simulink subsystem "station2a"  (R2024b)
settings: Solver=VariableStepAuto  StartTime=0.0  StopTime=10.0  RelTol=1e-3
undefined symbols (not defined in the file): DiscIntNeverNeededParam, h, R3, ResistanceM, Rt4, Ts, Zm
libraries: ee_lib x105, nesl_utility x83, fl_lib x73, simulink x6, simetran x1, powerlib_extras x1
(part 2 of 4)

== system station2a/Filters 60Hz4 ==
  s : Inport
  Circuit Breaker (Three-Phase) : ee_lib/Switches & Breakers/Circuit Breaker (Three-Phase)  R_closed=0.001 Ohm  G_open=1e-6 1/Ohm  threshold=0.5 V  breaker_behavior=ee.enum.switches.breakerBehavior.zeroCrossingEnable
      settings: InternalSimscapePortConfiguration="{\"Bottom\":[],\"Left\":[{\"id\":\"vT\",\"label\":\"vT\",\"type\":\"input\"},{\"id\":\"N1\",\"label\":\"~1\",\"type\":\"foundation.electrical.three_phase\"}],\"Right\":[{\"id\":\"N2\",\"label\":\"~2\",\"type\":\"foundation.electrical.three_phase\"}],\"Top\":[]}"
  Constant : Constant
  Electrical Reference : fl_lib/Electrical/Electrical Elements/Electrical Reference
  Simulink-PS Converter : nesl_utility/Simulink-PS Converter  PhysicalDomain=network_engine_domain  SubClassName=ps_input  LeftPortType=input  RightPortType=output  PseudoPeriodic=off  Frequencies=[]  NoiseDistribution=none  NoiseParameters=[]  Unit=1  AffineConversion=off  FilteringAndDerivatives=provide  SimscapeFilterOrder=1  InputFilterTimeConstant=0.001  UdotUserProvided=0
  Sum : Sum  Inputs=|-+
  Wye-Connected Load : ee_lib/Passive/RLC Assemblies/Wye-Connected Load  port_option=ee.enum.threePhasePort.composite  parameterization=ee.enum.rlc.parameterization.ratedpower  component_structure=ee.enum.rlc.structure.R  component_structure_PQ=ee.enum.rlc.structure.C  R=1 Ohm  L=1e-3 H  C=1e-6 F  VRated=345e3 V  FRated=50 Hz  P=1e3 W  Qpos=1e2 A*V  Qneg=-150e6/4 A*V  R_parasitic=1e-6 Ohm  G_parasitic=1e-6 1/Ohm  R_parasitic_PQ=0 Ohm  G_parasitic_PQ=1e-6 1/Ohm  Vmag0=500e3 V  Vang0=0 deg  Freq0=60 Hz  IL_specify=off  IL_priority=High  IL=[0, 0, 0] A  IL_nominal_specify=off  IL_nominal_value=1  IL_nominal_unit=A  VC_specify=off  VC_priority=High  VC=[0, 0, 0] V  VC_nominal_specify=off  VC_nominal_value=1  VC_nominal_unit=V
  high-pass filter : ee_lib/Passive/Passive Harmonic Filter (Three-Phase)  QRated=150e6/4 A*V  VRated=345e3 V  FRated=50 Hz  qfactor=3  type_option=ee.enum.filtertype.HPsecondorder  connection_option=ee.enum.filterconnection.Yg  ftuned=24 * 24 Hz  ftuned1=7 * 60 Hz  ftuned2=11 * 60 Hz  I_specify=off  I_priority=None  I=[0, 0, 0] A  I_nominal_specify=off  I_nominal_value=1  I_nominal_unit=A  V_specify=off  V_priority=None  V=[0, 0, 0] V  V_nominal_specify=off  V_nominal_value=1  V_nominal_unit=V
      settings: InternalSimscapePortConfiguration="{\"Bottom\":[],\"Left\":[{\"id\":\"N\",\"label\":\"~\",\"type\":\"foundation.electrical.three_phase\"}],\"Right\":[],\"Top\":[]}"
  tuned flter 11th : ee_lib/Passive/Passive Harmonic Filter (Three-Phase)  QRated=150e6/4 A*V  VRated=345e3 V  FRated=50 Hz  qfactor=100  type_option=ee.enum.filtertype.BPsingle  connection_option=ee.enum.filterconnection.Yg  ftuned=11 * 50 Hz  ftuned1=7 * 60 Hz  ftuned2=11 * 60 Hz  I_specify=off  I_priority=None  I=[0, 0, 0] A  I_nominal_specify=off  I_nominal_value=1  I_nominal_unit=A  V_specify=off  V_priority=None  V=[0, 0, 0] V  V_nominal_specify=off  V_nominal_value=1  V_nominal_unit=V
      settings: InternalSimscapePortConfiguration="{\"Bottom\":[],\"Left\":[{\"id\":\"N\",\"label\":\"~\",\"type\":\"foundation.electrical.three_phase\"}],\"Right\":[],\"Top\":[]}"
  tuned flter 13th : ee_lib/Passive/Passive Harmonic Filter (Three-Phase)  QRated=150e6/4 A*V  VRated=345e3 V  FRated=50 Hz  qfactor=100  type_option=ee.enum.filtertype.BPsingle  connection_option=ee.enum.filterconnection.Yg  ftuned=13 * 50 Hz  ftuned1=7 * 60 Hz  ftuned2=11 * 60 Hz  I_specify=off  I_priority=None  I=[0, 0, 0] A  I_nominal_specify=off  I_nominal_value=1  I_nominal_unit=A  V_specify=off  V_priority=None  V=[0, 0, 0] V  V_nominal_specify=off  V_nominal_value=1  V_nominal_unit=V
      settings: InternalSimscapePortConfiguration="{\"Bottom\":[],\"Left\":[{\"id\":\"N\",\"label\":\"~\",\"type\":\"foundation.electrical.three_phase\"}],\"Right\":[],\"Top\":[]}"
  abc : PMIOPort  Side=Right
  wires:
  s/1 -> Sum/1
  Constant/1 -> Sum/2
  Sum/1 -> Simulink-PS Converter/1
  connections:
  Electrical Reference/LConn1 -- Wye-Connected Load/RConn1
  Wye-Connected Load/LConn1 -- high-pass filter/LConn1 -- tuned flter 13th/LConn1 -- Circuit Breaker (Three-Phase)/LConn2 -- tuned flter 11th/LConn1
  Circuit Breaker (Three-Phase)/RConn1 -- abc/RConn1
  Simulink-PS Converter/RConn1 -- Circuit Breaker (Three-Phase)/LConn1

== system station2a/Filters 60Hz5 ==
  s : Inport
  Circuit Breaker (Three-Phase) : ee_lib/Switches & Breakers/Circuit Breaker (Three-Phase)  R_closed=0.001 Ohm  G_open=1e-6 1/Ohm  threshold=0.5 V  breaker_behavior=ee.enum.switches.breakerBehavior.zeroCrossingEnable
      settings: InternalSimscapePortConfiguration="{\"Bottom\":[],\"Left\":[{\"id\":\"vT\",\"label\":\"vT\",\"type\":\"input\"},{\"id\":\"N1\",\"label\":\"~1\",\"type\":\"foundation.electrical.three_phase\"}],\"Right\":[{\"id\":\"N2\",\"label\":\"~2\",\"type\":\"foundation.electrical.three_phase\"}],\"Top\":[]}"
  Constant : Constant
  Electrical Reference : fl_lib/Electrical/Electrical Elements/Electrical Reference
  Simulink-PS Converter : nesl_utility/Simulink-PS Converter  PhysicalDomain=network_engine_domain  SubClassName=ps_input  LeftPortType=input  RightPortType=output  PseudoPeriodic=off  Frequencies=[]  NoiseDistribution=none  NoiseParameters=[]  Unit=1  AffineConversion=off  FilteringAndDerivatives=provide  SimscapeFilterOrder=1  InputFilterTimeConstant=0.001  UdotUserProvided=0
  Sum : Sum  Inputs=|-+
  Wye-Connected Load : ee_lib/Passive/RLC Assemblies/Wye-Connected Load  port_option=ee.enum.threePhasePort.composite  parameterization=ee.enum.rlc.parameterization.ratedpower  component_structure=ee.enum.rlc.structure.R  component_structure_PQ=ee.enum.rlc.structure.C  R=1 Ohm  L=1e-3 H  C=1e-6 F  VRated=345e3 V  FRated=50 Hz  P=1e3 W  Qpos=1e2 A*V  Qneg=-150e6/4 A*V  R_parasitic=1e-6 Ohm  G_parasitic=1e-6 1/Ohm  R_parasitic_PQ=0 Ohm  G_parasitic_PQ=1e-6 1/Ohm  Vmag0=500e3 V  Vang0=0 deg  Freq0=60 Hz  IL_specify=off  IL_priority=High  IL=[0, 0, 0] A  IL_nominal_specify=off  IL_nominal_value=1  IL_nominal_unit=A  VC_specify=off  VC_priority=High  VC=[0, 0, 0] V  VC_nominal_specify=off  VC_nominal_value=1  VC_nominal_unit=V
  high-pass filter : ee_lib/Passive/Passive Harmonic Filter (Three-Phase)  QRated=150e6/4 A*V  VRated=345e3 V  FRated=50 Hz  qfactor=3  type_option=ee.enum.filtertype.HPsecondorder  connection_option=ee.enum.filterconnection.Yg  ftuned=24 * 24 Hz  ftuned1=7 * 60 Hz  ftuned2=11 * 60 Hz  I_specify=off  I_priority=None  I=[0, 0, 0] A  I_nominal_specify=off  I_nominal_value=1  I_nominal_unit=A  V_specify=off  V_priority=None  V=[0, 0, 0] V  V_nominal_specify=off  V_nominal_value=1  V_nominal_unit=V
      settings: InternalSimscapePortConfiguration="{\"Bottom\":[],\"Left\":[{\"id\":\"N\",\"label\":\"~\",\"type\":\"foundation.electrical.three_phase\"}],\"Right\":[],\"Top\":[]}"
  tuned flter 11th : ee_lib/Passive/Passive Harmonic Filter (Three-Phase)  QRated=150e6/4 A*V  VRated=345e3 V  FRated=50 Hz  qfactor=100  type_option=ee.enum.filtertype.BPsingle  connection_option=ee.enum.filterconnection.Yg  ftuned=11 * 50 Hz  ftuned1=7 * 60 Hz  ftuned2=11 * 60 Hz  I_specify=off  I_priority=None  I=[0, 0, 0] A  I_nominal_specify=off  I_nominal_value=1  I_nominal_unit=A  V_specify=off  V_priority=None  V=[0, 0, 0] V  V_nominal_specify=off  V_nominal_value=1  V_nominal_unit=V
      settings: InternalSimscapePortConfiguration="{\"Bottom\":[],\"Left\":[{\"id\":\"N\",\"label\":\"~\",\"type\":\"foundation.electrical.three_phase\"}],\"Right\":[],\"Top\":[]}"
  tuned flter 13th : ee_lib/Passive/Passive Harmonic Filter (Three-Phase)  QRated=150e6/4 A*V  VRated=345e3 V  FRated=50 Hz  qfactor=100  type_option=ee.enum.filtertype.BPsingle  connection_option=ee.enum.filterconnection.Yg  ftuned=13 * 50 Hz  ftuned1=7 * 60 Hz  ftuned2=11 * 60 Hz  I_specify=off  I_priority=None  I=[0, 0, 0] A  I_nominal_specify=off  I_nominal_value=1  I_nominal_unit=A  V_specify=off  V_priority=None  V=[0, 0, 0] V  V_nominal_specify=off  V_nominal_value=1  V_nominal_unit=V
      settings: InternalSimscapePortConfiguration="{\"Bottom\":[],\"Left\":[{\"id\":\"N\",\"label\":\"~\",\"type\":\"foundation.electrical.three_phase\"}],\"Right\":[],\"Top\":[]}"
  abc : PMIOPort  Side=Right
  wires:
  Sum/1 -> Simulink-PS Converter/1
  Constant/1 -> Sum/2
  s/1 -> Sum/1
  connections:
  Simulink-PS Converter/RConn1 -- Circuit Breaker (Three-Phase)/LConn1
  Circuit Breaker (Three-Phase)/RConn1 -- abc/RConn1
  tuned flter 11th/LConn1 -- Circuit Breaker (Three-Phase)/LConn2 -- tuned flter 13th/LConn1 -- high-pass filter/LConn1 -- Wye-Connected Load/LConn1
  Electrical Reference/LConn1 -- Wye-Connected Load/RConn1

== system station2a/Filters 60Hz6 ==
  s : Inport
  Circuit Breaker (Three-Phase) : ee_lib/Switches & Breakers/Circuit Breaker (Three-Phase)  R_closed=0.001 Ohm  G_open=1e-6 1/Ohm  threshold=0.5 V  breaker_behavior=ee.enum.switches.breakerBehavior.zeroCrossingEnable
      settings: InternalSimscapePortConfiguration="{\"Bottom\":[],\"Left\":[{\"id\":\"vT\",\"label\":\"vT\",\"type\":\"input\"},{\"id\":\"N1\",\"label\":\"~1\",\"type\":\"foundation.electrical.three_phase\"}],\"Right\":[{\"id\":\"N2\",\"label\":\"~2\",\"type\":\"foundation.electrical.three_phase\"}],\"Top\":[]}"
  Constant : Constant
  Electrical Reference : fl_lib/Electrical/Electrical Elements/Electrical Reference
  Simulink-PS Converter : nesl_utility/Simulink-PS Converter  PhysicalDomain=network_engine_domain  SubClassName=ps_input  LeftPortType=input  RightPortType=output  PseudoPeriodic=off  Frequencies=[]  NoiseDistribution=none  NoiseParameters=[]  Unit=1  AffineConversion=off  FilteringAndDerivatives=provide  SimscapeFilterOrder=1  InputFilterTimeConstant=0.001  UdotUserProvided=0
  Sum : Sum  Inputs=|-+
  Wye-Connected Load : ee_lib/Passive/RLC Assemblies/Wye-Connected Load  port_option=ee.enum.threePhasePort.composite  parameterization=ee.enum.rlc.parameterization.ratedpower  component_structure=ee.enum.rlc.structure.R  component_structure_PQ=ee.enum.rlc.structure.C  R=1 Ohm  L=1e-3 H  C=1e-6 F  VRated=345e3 V  FRated=50 Hz  P=1e3 W  Qpos=1e2 A*V  Qneg=-150e6/4 A*V  R_parasitic=1e-6 Ohm  G_parasitic=1e-6 1/Ohm  R_parasitic_PQ=0 Ohm  G_parasitic_PQ=1e-6 1/Ohm  Vmag0=500e3 V  Vang0=0 deg  Freq0=60 Hz  IL_specify=off  IL_priority=High  IL=[0, 0, 0] A  IL_nominal_specify=off  IL_nominal_value=1  IL_nominal_unit=A  VC_specify=off  VC_priority=High  VC=[0, 0, 0] V  VC_nominal_specify=off  VC_nominal_value=1  VC_nominal_unit=V
  high-pass filter : ee_lib/Passive/Passive Harmonic Filter (Three-Phase)  QRated=150e6/4 A*V  VRated=345e3 V  FRated=50 Hz  qfactor=3  type_option=ee.enum.filtertype.HPsecondorder  connection_option=ee.enum.filterconnection.Yg  ftuned=24 * 24 Hz  ftuned1=7 * 60 Hz  ftuned2=11 * 60 Hz  I_specify=off  I_priority=None  I=[0, 0, 0] A  I_nominal_specify=off  I_nominal_value=1  I_nominal_unit=A  V_specify=off  V_priority=None  V=[0, 0, 0] V  V_nominal_specify=off  V_nominal_value=1  V_nominal_unit=V
      settings: InternalSimscapePortConfiguration="{\"Bottom\":[],\"Left\":[{\"id\":\"N\",\"label\":\"~\",\"type\":\"foundation.electrical.three_phase\"}],\"Right\":[],\"Top\":[]}"
  tuned flter 11th : ee_lib/Passive/Passive Harmonic Filter (Three-Phase)  QRated=150e6/4 A*V  VRated=345e3 V  FRated=50 Hz  qfactor=100  type_option=ee.enum.filtertype.BPsingle  connection_option=ee.enum.filterconnection.Yg  ftuned=11 * 50 Hz  ftuned1=7 * 60 Hz  ftuned2=11 * 60 Hz  I_specify=off  I_priority=None  I=[0, 0, 0] A  I_nominal_specify=off  I_nominal_value=1  I_nominal_unit=A  V_specify=off  V_priority=None  V=[0, 0, 0] V  V_nominal_specify=off  V_nominal_value=1  V_nominal_unit=V
      settings: InternalSimscapePortConfiguration="{\"Bottom\":[],\"Left\":[{\"id\":\"N\",\"label\":\"~\",\"type\":\"foundation.electrical.three_phase\"}],\"Right\":[],\"Top\":[]}"
  tuned flter 13th : ee_lib/Passive/Passive Harmonic Filter (Three-Phase)  QRated=150e6/4 A*V  VRated=345e3 V  FRated=50 Hz  qfactor=100  type_option=ee.enum.filtertype.BPsingle  connection_option=ee.enum.filterconnection.Yg  ftuned=13 * 50 Hz  ftuned1=7 * 60 Hz  ftuned2=11 * 60 Hz  I_specify=off  I_priority=None  I=[0, 0, 0] A  I_nominal_specify=off  I_nominal_value=1  I_nominal_unit=A  V_specify=off  V_priority=None  V=[0, 0, 0] V  V_nominal_specify=off  V_nominal_value=1  V_nominal_unit=V
      settings: InternalSimscapePortConfiguration="{\"Bottom\":[],\"Left\":[{\"id\":\"N\",\"label\":\"~\",\"type\":\"foundation.electrical.three_phase\"}],\"Right\":[],\"Top\":[]}"
  abc : PMIOPort  Side=Right
  wires:
  s/1 -> Sum/1
  Constant/1 -> Sum/2
  Sum/1 -> Simulink-PS Converter/1
  connections:
  Electrical Reference/LConn1 -- Wye-Connected Load/RConn1
  Wye-Connected Load/LConn1 -- high-pass filter/LConn1 -- tuned flter 13th/LConn1 -- Circuit Breaker (Three-Phase)/LConn2 -- tuned flter 11th/LConn1
  Circuit Breaker (Three-Phase)/RConn1 -- abc/RConn1
  Simulink-PS Converter/RConn1 -- Circuit Breaker (Three-Phase)/LConn1

== system station2a/Filters 60Hz7 ==
  s : Inport
  Circuit Breaker (Three-Phase) : ee_lib/Switches & Breakers/Circuit Breaker (Three-Phase)  R_closed=0.001 Ohm  G_open=1e-6 1/Ohm  threshold=0.5 V  breaker_behavior=ee.enum.switches.breakerBehavior.zeroCrossingEnable
      settings: InternalSimscapePortConfiguration="{\"Bottom\":[],\"Left\":[{\"id\":\"vT\",\"label\":\"vT\",\"type\":\"input\"},{\"id\":\"N1\",\"label\":\"~1\",\"type\":\"foundation.electrical.three_phase\"}],\"Right\":[{\"id\":\"N2\",\"label\":\"~2\",\"type\":\"foundation.electrical.three_phase\"}],\"Top\":[]}"
  Constant : Constant
  Electrical Reference : fl_lib/Electrical/Electrical Elements/Electrical Reference
  Simulink-PS Converter : nesl_utility/Simulink-PS Converter  PhysicalDomain=network_engine_domain  SubClassName=ps_input  LeftPortType=input  RightPortType=output  PseudoPeriodic=off  Frequencies=[]  NoiseDistribution=none  NoiseParameters=[]  Unit=1  AffineConversion=off  FilteringAndDerivatives=provide  SimscapeFilterOrder=1  InputFilterTimeConstant=0.001  UdotUserProvided=0
  Sum : Sum  Inputs=|-+
  Wye-Connected Load : ee_lib/Passive/RLC Assemblies/Wye-Connected Load  port_option=ee.enum.threePhasePort.composite  parameterization=ee.enum.rlc.parameterization.ratedpower  component_structure=ee.enum.rlc.structure.R  component_structure_PQ=ee.enum.rlc.structure.C  R=1 Ohm  L=1e-3 H  C=1e-6 F  VRated=345e3 V  FRated=50 Hz  P=1e3 W  Qpos=1e2 A*V  Qneg=-150e6/4 A*V  R_parasitic=1e-6 Ohm  G_parasitic=1e-6 1/Ohm  R_parasitic_PQ=0 Ohm  G_parasitic_PQ=1e-6 1/Ohm  Vmag0=500e3 V  Vang0=0 deg  Freq0=60 Hz  IL_specify=off  IL_priority=High  IL=[0, 0, 0] A  IL_nominal_specify=off  IL_nominal_value=1  IL_nominal_unit=A  VC_specify=off  VC_priority=High  VC=[0, 0, 0] V  VC_nominal_specify=off  VC_nominal_value=1  VC_nominal_unit=V
  high-pass filter : ee_lib/Passive/Passive Harmonic Filter (Three-Phase)  QRated=150e6/4 A*V  VRated=345e3 V  FRated=50 Hz  qfactor=3  type_option=ee.enum.filtertype.HPsecondorder  connection_option=ee.enum.filterconnection.Yg  ftuned=24 * 24 Hz  ftuned1=7 * 60 Hz  ftuned2=11 * 60 Hz  I_specify=off  I_priority=None  I=[0, 0, 0] A  I_nominal_specify=off  I_nominal_value=1  I_nominal_unit=A  V_specify=off  V_priority=None  V=[0, 0, 0] V  V_nominal_specify=off  V_nominal_value=1  V_nominal_unit=V
      settings: InternalSimscapePortConfiguration="{\"Bottom\":[],\"Left\":[{\"id\":\"N\",\"label\":\"~\",\"type\":\"foundation.electrical.three_phase\"}],\"Right\":[],\"Top\":[]}"
  tuned flter 11th : ee_lib/Passive/Passive Harmonic Filter (Three-Phase)  QRated=150e6/4 A*V  VRated=345e3 V  FRated=50 Hz  qfactor=100  type_option=ee.enum.filtertype.BPsingle  connection_option=ee.enum.filterconnection.Yg  ftuned=11 * 50 Hz  ftuned1=7 * 60 Hz  ftuned2=11 * 60 Hz  I_specify=off  I_priority=None  I=[0, 0, 0] A  I_nominal_specify=off  I_nominal_value=1  I_nominal_unit=A  V_specify=off  V_priority=None  V=[0, 0, 0] V  V_nominal_specify=off  V_nominal_value=1  V_nominal_unit=V
      settings: InternalSimscapePortConfiguration="{\"Bottom\":[],\"Left\":[{\"id\":\"N\",\"label\":\"~\",\"type\":\"foundation.electrical.three_phase\"}],\"Right\":[],\"Top\":[]}"
  tuned flter 13th : ee_lib/Passive/Passive Harmonic Filter (Three-Phase)  QRated=150e6/4 A*V  VRated=345e3 V  FRated=50 Hz  qfactor=100  type_option=ee.enum.filtertype.BPsingle  connection_option=ee.enum.filterconnection.Yg  ftuned=13 * 50 Hz  ftuned1=7 * 60 Hz  ftuned2=11 * 60 Hz  I_specify=off  I_priority=None  I=[0, 0, 0] A  I_nominal_specify=off  I_nominal_value=1  I_nominal_unit=A  V_specify=off  V_priority=None  V=[0, 0, 0] V  V_nominal_specify=off  V_nominal_value=1  V_nominal_unit=V
      settings: InternalSimscapePortConfiguration="{\"Bottom\":[],\"Left\":[{\"id\":\"N\",\"label\":\"~\",\"type\":\"foundation.electrical.three_phase\"}],\"Right\":[],\"Top\":[]}"
  abc : PMIOPort  Side=Right
  wires:
  Sum/1 -> Simulink-PS Converter/1
  Constant/1 -> Sum/2
  s/1 -> Sum/1
  connections:
  Simulink-PS Converter/RConn1 -- Circuit Breaker (Three-Phase)/LConn1
  Circuit Breaker (Three-Phase)/RConn1 -- abc/RConn1
  tuned flter 11th/LConn1 -- Circuit Breaker (Three-Phase)/LConn2 -- tuned flter 13th/LConn1 -- high-pass filter/LConn1 -- Wye-Connected Load/LConn1
  Electrical Reference/LConn1 -- Wye-Connected Load/RConn1

== system station2a/Filters 60Hz8 ==
  s : Inport
  Circuit Breaker (Three-Phase) : ee_lib/Switches & Breakers/Circuit Breaker (Three-Phase)  R_closed=0.001 Ohm  G_open=1e-6 1/Ohm  threshold=0.5 V  breaker_behavior=ee.enum.switches.breakerBehavior.zeroCrossingEnable
      settings: InternalSimscapePortConfiguration="{\"Bottom\":[],\"Left\":[{\"id\":\"vT\",\"label\":\"vT\",\"type\":\"input\"},{\"id\":\"N1\",\"label\":\"~1\",\"type\":\"foundation.electrical.three_phase\"}],\"Right\":[{\"id\":\"N2\",\"label\":\"~2\",\"type\":\"foundation.electrical.three_phase\"}],\"Top\":[]}"
  Constant : Constant
  Electrical Reference : fl_lib/Electrical/Electrical Elements/Electrical Reference
  Simulink-PS Converter : nesl_utility/Simulink-PS Converter  PhysicalDomain=network_engine_domain  SubClassName=ps_input  LeftPortType=input  RightPortType=output  PseudoPeriodic=off  Frequencies=[]  NoiseDistribution=none  NoiseParameters=[]  Unit=1  AffineConversion=off  FilteringAndDerivatives=provide  SimscapeFilterOrder=1  InputFilterTimeConstant=0.001  UdotUserProvided=0
  Sum : Sum  Inputs=|-+
  Wye-Connected Load : ee_lib/Passive/RLC Assemblies/Wye-Connected Load  port_option=ee.enum.threePhasePort.composite  parameterization=ee.enum.rlc.parameterization.ratedpower  component_structure=ee.enum.rlc.structure.R  component_structure_PQ=ee.enum.rlc.structure.C  R=1 Ohm  L=1e-3 H  C=1e-6 F  VRated=345e3 V  FRated=50 Hz  P=1e3 W  Qpos=1e2 A*V  Qneg=-150e6/4 A*V  R_parasitic=1e-6 Ohm  G_parasitic=1e-6 1/Ohm  R_parasitic_PQ=0 Ohm  G_parasitic_PQ=1e-6 1/Ohm  Vmag0=500e3 V  Vang0=0 deg  Freq0=60 Hz  IL_specify=off  IL_priority=High  IL=[0, 0, 0] A  IL_nominal_specify=off  IL_nominal_value=1  IL_nominal_unit=A  VC_specify=off  VC_priority=High  VC=[0, 0, 0] V  VC_nominal_specify=off  VC_nominal_value=1  VC_nominal_unit=V
  high-pass filter : ee_lib/Passive/Passive Harmonic Filter (Three-Phase)  QRated=150e6/4 A*V  VRated=345e3 V  FRated=50 Hz  qfactor=3  type_option=ee.enum.filtertype.HPsecondorder  connection_option=ee.enum.filterconnection.Yg  ftuned=24 * 24 Hz  ftuned1=7 * 60 Hz  ftuned2=11 * 60 Hz  I_specify=off  I_priority=None  I=[0, 0, 0] A  I_nominal_specify=off  I_nominal_value=1  I_nominal_unit=A  V_specify=off  V_priority=None  V=[0, 0, 0] V  V_nominal_specify=off  V_nominal_value=1  V_nominal_unit=V
      settings: InternalSimscapePortConfiguration="{\"Bottom\":[],\"Left\":[{\"id\":\"N\",\"label\":\"~\",\"type\":\"foundation.electrical.three_phase\"}],\"Right\":[],\"Top\":[]}"
  tuned flter 11th : ee_lib/Passive/Passive Harmonic Filter (Three-Phase)  QRated=150e6/4 A*V  VRated=345e3 V  FRated=50 Hz  qfactor=100  type_option=ee.enum.filtertype.BPsingle  connection_option=ee.enum.filterconnection.Yg  ftuned=11 * 50 Hz  ftuned1=7 * 60 Hz  ftuned2=11 * 60 Hz  I_specify=off  I_priority=None  I=[0, 0, 0] A  I_nominal_specify=off  I_nominal_value=1  I_nominal_unit=A  V_specify=off  V_priority=None  V=[0, 0, 0] V  V_nominal_specify=off  V_nominal_value=1  V_nominal_unit=V
      settings: InternalSimscapePortConfiguration="{\"Bottom\":[],\"Left\":[{\"id\":\"N\",\"label\":\"~\",\"type\":\"foundation.electrical.three_phase\"}],\"Right\":[],\"Top\":[]}"
  tuned flter 13th : ee_lib/Passive/Passive Harmonic Filter (Three-Phase)  QRated=150e6/4 A*V  VRated=345e3 V  FRated=50 Hz  qfactor=100  type_option=ee.enum.filtertype.BPsingle  connection_option=ee.enum.filterconnection.Yg  ftuned=13 * 50 Hz  ftuned1=7 * 60 Hz  ftuned2=11 * 60 Hz  I_specify=off  I_priority=None  I=[0, 0, 0] A  I_nominal_specify=off  I_nominal_value=1  I_nominal_unit=A  V_specify=off  V_priority=None  V=[0, 0, 0] V  V_nominal_specify=off  V_nominal_value=1  V_nominal_unit=V
      settings: InternalSimscapePortConfiguration="{\"Bottom\":[],\"Left\":[{\"id\":\"N\",\"label\":\"~\",\"type\":\"foundation.electrical.three_phase\"}],\"Right\":[],\"Top\":[]}"
  abc : PMIOPort  Side=Right
  wires:
  Sum/1 -> Simulink-PS Converter/1
  Constant/1 -> Sum/2
  s/1 -> Sum/1
  connections:
  Simulink-PS Converter/RConn1 -- Circuit Breaker (Three-Phase)/LConn1
  Circuit Breaker (Three-Phase)/RConn1 -- abc/RConn1
  tuned flter 11th/LConn1 -- Circuit Breaker (Three-Phase)/LConn2 -- tuned flter 13th/LConn1 -- high-pass filter/LConn1 -- Wye-Connected Load/LConn1
  Electrical Reference/LConn1 -- Wye-Connected Load/RConn1

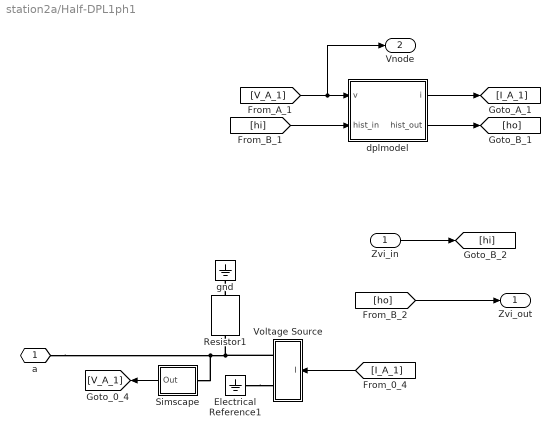
== system station2a/Half-DPL1ph1 ==
  Zvi_in : Inport
  Electrical Reference1 : fl_lib/Electrical/Electrical Elements/Electrical Reference
  Resistor1 : ee_lib/Passive/Resistor  R=ResistanceM(1,1) Ohm  enable_R_tol=ee.enum.toleranceApplication.none  R_tol=5  tol_distribution=ee.enum.toleranceDistribution.uniform  nSigma=4  enable_operating_limits=ee.enum.enable.no  operating_limit_action=ee.enum.passive.reportOpLim.warn  power_rating=1 W  max_working_voltage=100 V  noise_mode=ee.enum.sources.noise.Disabled  Tdevice=25 degC  sample_time=1e-3 s  repeatability=ee.enum.ic.repeatability.notRepeatable  user_seed=0  auto_seed=2070268988  fault_action=simscape.enum.assert.action.none  t_fault=1 s  power_derating_T1=70 degC  power_derating_T2=155 degC  operating_temperature_range_vec=[-50, 150] degC  alpha=3.93e-3 1/K  Tmeas=25 degC  thermal_mass=100 J/K  temperature_specify=off  temperature_priority=High  temperature=298.15 K  temperature_nominal_specify=off  temperature_nominal_value=1  temperature_nominal_unit=K
  Simscape : Subsystem
      mask Display: disp('V')
  Voltage Source : Subsystem
  dplmodel : Subsystem
  gnd : fl_lib/Electrical/Electrical Elements/Electrical Reference
  a : PMIOPort  Side=Left
  Zvi_out : Outport  VectorParamsAs1DForOutWhenUnconnected=off
  Vnode : Outport  Port=2  VectorParamsAs1DForOutWhenUnconnected=off
  wires:
  [ho] -> Zvi_out/1
  dplmodel/1(i) -> [I_A_1]
  [V_A_1] -> Vnode/1, dplmodel/1(v)
  Zvi_in/1 -> [hi]
  [hi] -> dplmodel/2(hist_in)
  dplmodel/2(hist_out) -> [ho]
  Simscape/1(Out) -> [V_A_1]
  [I_A_1] -> Voltage Source/1(I)
  connections:
  a/RConn1 -- Simscape/LConn1 -- Voltage Source/RConn1 -- Resistor1/RConn1
  Resistor1/LConn1 -- gnd/LConn1
  Electrical Reference1/LConn1 -- Voltage Source/RConn2

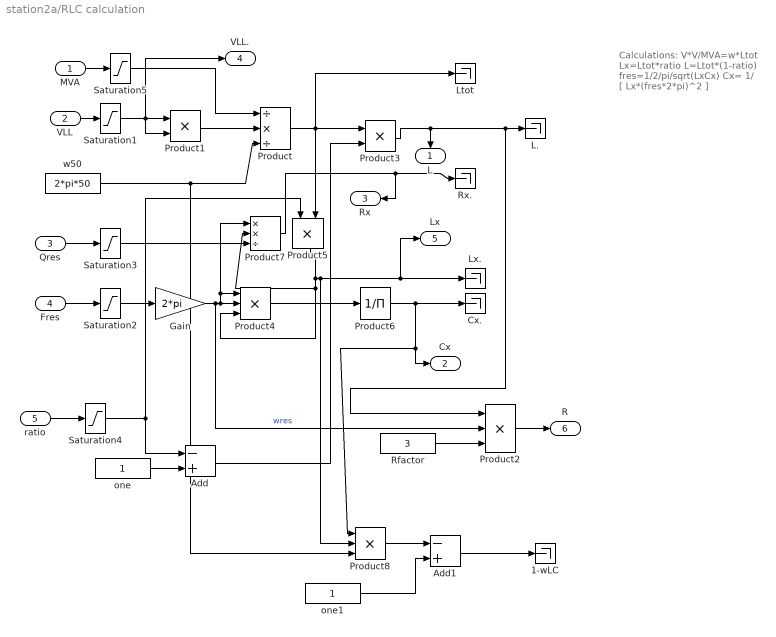
== system station2a/RLC calculation ==
  note: Calculations:
      |
      | V*V/MVA=w*Ltot
      | Lx=Ltot*ratio
      | L=Ltot*(1-ratio)
      |
      |
      | fres=1/2/pi/sqrt(LxCx)
      |
      | Cx= 1/ [ Lx*(fres*2*pi)^2 ]
  MVA : Inport
  VLL : Inport  Port=2
  Qres : Inport  Port=3
  Fres : Inport  Port=4
  ratio : Inport  Port=5
  1-wLC : Terminator
  Add : Sum  Inputs=-+
  Add1 : Sum  Inputs=-+
  Cx. : Terminator
  Gain : Gain  Gain=2*pi
  L. : Terminator
  Ltot : Terminator
  Lx. : Terminator
  Product : Product  Inputs=/*/  RndMeth=Zero
  Product1 : Product  RndMeth=Zero
  Product2 : Product  Inputs=3  RndMeth=Zero
  Product3 : Product  RndMeth=Zero
  Product4 : Product  Inputs=3  RndMeth=Zero
  Product5 : Product  RndMeth=Zero
  Product6 : Product  Inputs=/  RndMeth=Zero
  Product7 : Product  Inputs=**/  RndMeth=Zero
  Product8 : Product  Inputs=3  RndMeth=Zero
  Rfactor : Constant  Value=3
  Rx. : Terminator
  Saturation1 : Saturate  UpperLimit=inf  LowerLimit=1
  Saturation2 : Saturate  UpperLimit=inf  LowerLimit=1
  Saturation3 : Saturate  UpperLimit=inf  LowerLimit=0.1
  Saturation4 : Saturate  UpperLimit=inf  LowerLimit=0.001
  Saturation5 : Saturate  UpperLimit=inf  LowerLimit=1
  one : Constant
  one1 : Constant
  w50 : Constant  Value=2*pi*50
  L : Outport
  Cx : Outport  Port=2
  Rx : Outport  Port=3
  VLL. : Outport  Port=4
  Lx : Outport  Port=5
  R : Outport  Port=6
  wires:
  Add1/1 -> 1-wLC/1
  one1/1 -> Add1/2
  Product8/1 -> Add1/1
  Saturation5/1 -> Product/1
  Saturation4/1 -> Add/1, Product5/1
  Saturation3/1 -> Product7/3
  Saturation2/1 -> Gain/1
  Saturation1/1 -> VLL./1, Product1/1, Product1/2
  Add/1 -> Product3/2
  one/1 -> Add/2
  ratio/1 -> Saturation4/1
  Product2/1 -> R/1
  Rfactor/1 -> Product2/3
  Fres/1 -> Saturation2/1
  Qres/1 -> Saturation3/1
  MVA/1 -> Saturation5/1
  VLL/1 -> Saturation1/1
  Product7/1 -> Rx/1, Rx./1
  Product6/1 -> Product8/1, Cx/1, Cx./1
  Product4/1 -> Product6/1
  Product5/1 -> Product8/2, Lx/1, Lx./1, Product4/3, Product7/2
  Gain/1 -> Product2/2, Product4/2, Product4/1, Product7/1  "wres"
  w50/1 -> Product8/3, Product/3
  Product3/1 -> Product2/1, L./1, L/1
  Product/1 -> Product5/2, Product3/1, Ltot/1
  Product1/1 -> Product/2

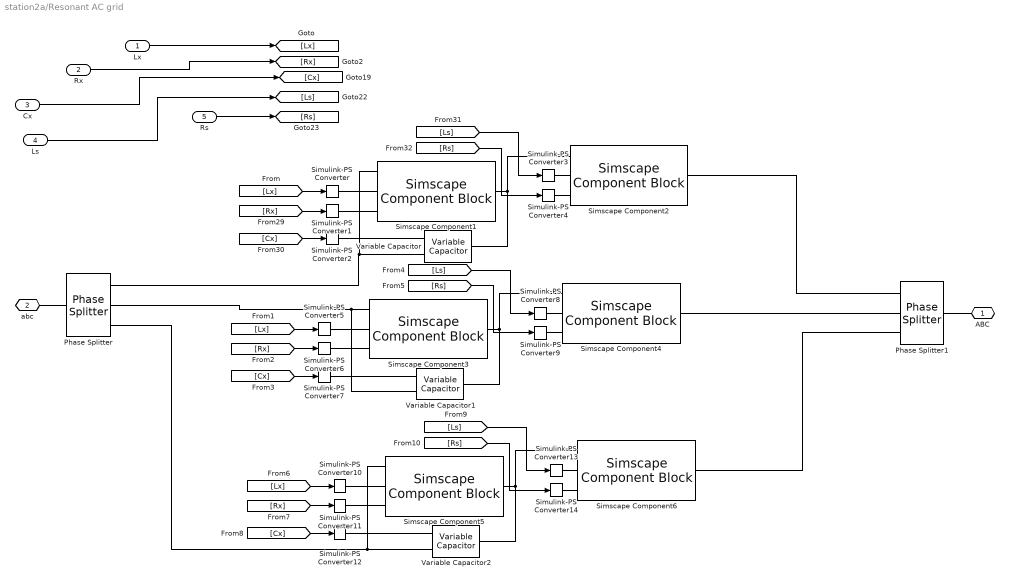
== system station2a/Resonant AC grid ==
  Lx : Inport
  Rx : Inport  Port=2
  Cx : Inport  Port=3
  Ls : Inport  Port=4
  Rs : Inport  Port=5
  Phase Splitter : ee_lib/Connectors & References/Phase Splitter
  Phase Splitter1 : ee_lib/Connectors & References/Phase Splitter
  Simscape Component1 : SimscapeComponentBlock  SourceFile=variableRL  ComponentPath=variableRL  ComponentVariants="[\"variableRL\"]"  ComponentVariantNames="[\"variableRL\"]"  ClassName=variableRL  SchemaVersion=1  g=1e-9 1/Ohm  typ=0  i_specify=off  i_priority=None  i=0 A  i_nominal_specify=off  i_nominal_value=1  i_nominal_unit=A  v_specify=off  v_priority=None  v=0 V  v_nominal_specify=off  v_nominal_value=1  v_nominal_unit=V  iL_specify=off  iL_priority=High  iL=0 A  iL_nominal_specify=off  iL_nominal_value=1  iL_nominal_unit=A
      settings: CopyFcn=simscape.engine.sli.internal.componentblockcallback(gcbh,'COPY')  PreCopyFcn=simscape.engine.sli.internal.componentblockcallback(gcbh,'PRECOPY')  PreDeleteFcn=simscape.engine.sli.internal.componentblockcallback(gcbh,'PREDELETE')  InternalSimscapePortConfiguration="{\"Bottom\":[],\"Left\":[{\"id\":\"p\",\"label\":\"+\",\"type\":\"foundation.electrical.electrical\"},{\"id\":\"L\",\"label\":\"L\",\"type\":\"input\"},{\"id\":\"R\",\"label\":\"R\",\"type\":\"input\"}],\"Right\":[{\"id\":\"n\",\"label\":\"-\",\"type\":\"foundation.electrical.electrical\"}],\"Top\":[]}"
      mask Type: simple Variable RL (series or parallel)
  Simscape Component2 : SimscapeComponentBlock  SourceFile=variableRL  ComponentPath=variableRL  ComponentVariants="[\"variableRL\"]"  ComponentVariantNames="[\"variableRL\"]"  ClassName=variableRL  SchemaVersion=1  g=1e-9 1/Ohm  typ=1  i_specify=off  i_priority=None  i=0 A  i_nominal_specify=off  i_nominal_value=1  i_nominal_unit=A  v_specify=off  v_priority=None  v=0 V  v_nominal_specify=off  v_nominal_value=1  v_nominal_unit=V  iL_specify=off  iL_priority=High  iL=0 A  iL_nominal_specify=off  iL_nominal_value=1  iL_nominal_unit=A
      settings: CopyFcn=simscape.engine.sli.internal.componentblockcallback(gcbh,'COPY')  PreCopyFcn=simscape.engine.sli.internal.componentblockcallback(gcbh,'PRECOPY')  PreDeleteFcn=simscape.engine.sli.internal.componentblockcallback(gcbh,'PREDELETE')  InternalSimscapePortConfiguration="{\"Bottom\":[],\"Left\":[{\"id\":\"p\",\"label\":\"+\",\"type\":\"foundation.electrical.electrical\"},{\"id\":\"L\",\"label\":\"L\",\"type\":\"input\"},{\"id\":\"R\",\"label\":\"R\",\"type\":\"input\"}],\"Right\":[{\"id\":\"n\",\"label\":\"-\",\"type\":\"foundation.electrical.electrical\"}],\"Top\":[]}"
      mask Type: simple Variable RL (series or parallel)
  Simscape Component3 : SimscapeComponentBlock  SourceFile=variableRL  ComponentPath=variableRL  ComponentVariants="[\"variableRL\"]"  ComponentVariantNames="[\"variableRL\"]"  ClassName=variableRL  SchemaVersion=1  g=1e-9 1/Ohm  typ=0  i_specify=off  i_priority=None  i=0 A  i_nominal_specify=off  i_nominal_value=1  i_nominal_unit=A  v_specify=off  v_priority=None  v=0 V  v_nominal_specify=off  v_nominal_value=1  v_nominal_unit=V  iL_specify=off  iL_priority=High  iL=0 A  iL_nominal_specify=off  iL_nominal_value=1  iL_nominal_unit=A
      settings: CopyFcn=simscape.engine.sli.internal.componentblockcallback(gcbh,'COPY')  PreCopyFcn=simscape.engine.sli.internal.componentblockcallback(gcbh,'PRECOPY')  PreDeleteFcn=simscape.engine.sli.internal.componentblockcallback(gcbh,'PREDELETE')  InternalSimscapePortConfiguration="{\"Bottom\":[],\"Left\":[{\"id\":\"p\",\"label\":\"+\",\"type\":\"foundation.electrical.electrical\"},{\"id\":\"L\",\"label\":\"L\",\"type\":\"input\"},{\"id\":\"R\",\"label\":\"R\",\"type\":\"input\"}],\"Right\":[{\"id\":\"n\",\"label\":\"-\",\"type\":\"foundation.electrical.electrical\"}],\"Top\":[]}"
      mask Type: simple Variable RL (series or parallel)
  Simscape Component4 : SimscapeComponentBlock  SourceFile=variableRL  ComponentPath=variableRL  ComponentVariants="[\"variableRL\"]"  ComponentVariantNames="[\"variableRL\"]"  ClassName=variableRL  SchemaVersion=1  g=1e-9 1/Ohm  typ=1  i_specify=off  i_priority=None  i=0 A  i_nominal_specify=off  i_nominal_value=1  i_nominal_unit=A  v_specify=off  v_priority=None  v=0 V  v_nominal_specify=off  v_nominal_value=1  v_nominal_unit=V  iL_specify=off  iL_priority=High  iL=0 A  iL_nominal_specify=off  iL_nominal_value=1  iL_nominal_unit=A
      settings: CopyFcn=simscape.engine.sli.internal.componentblockcallback(gcbh,'COPY')  PreCopyFcn=simscape.engine.sli.internal.componentblockcallback(gcbh,'PRECOPY')  PreDeleteFcn=simscape.engine.sli.internal.componentblockcallback(gcbh,'PREDELETE')  InternalSimscapePortConfiguration="{\"Bottom\":[],\"Left\":[{\"id\":\"p\",\"label\":\"+\",\"type\":\"foundation.electrical.electrical\"},{\"id\":\"L\",\"label\":\"L\",\"type\":\"input\"},{\"id\":\"R\",\"label\":\"R\",\"type\":\"input\"}],\"Right\":[{\"id\":\"n\",\"label\":\"-\",\"type\":\"foundation.electrical.electrical\"}],\"Top\":[]}"
      mask Type: simple Variable RL (series or parallel)
  Simscape Component5 : SimscapeComponentBlock  SourceFile=variableRL  ComponentPath=variableRL  ComponentVariants="[\"variableRL\"]"  ComponentVariantNames="[\"variableRL\"]"  ClassName=variableRL  SchemaVersion=1  g=1e-9 1/Ohm  typ=0  i_specify=off  i_priority=None  i=0 A  i_nominal_specify=off  i_nominal_value=1  i_nominal_unit=A  v_specify=off  v_priority=None  v=0 V  v_nominal_specify=off  v_nominal_value=1  v_nominal_unit=V  iL_specify=off  iL_priority=High  iL=0 A  iL_nominal_specify=off  iL_nominal_value=1  iL_nominal_unit=A
      settings: CopyFcn=simscape.engine.sli.internal.componentblockcallback(gcbh,'COPY')  PreCopyFcn=simscape.engine.sli.internal.componentblockcallback(gcbh,'PRECOPY')  PreDeleteFcn=simscape.engine.sli.internal.componentblockcallback(gcbh,'PREDELETE')  InternalSimscapePortConfiguration="{\"Bottom\":[],\"Left\":[{\"id\":\"p\",\"label\":\"+\",\"type\":\"foundation.electrical.electrical\"},{\"id\":\"L\",\"label\":\"L\",\"type\":\"input\"},{\"id\":\"R\",\"label\":\"R\",\"type\":\"input\"}],\"Right\":[{\"id\":\"n\",\"label\":\"-\",\"type\":\"foundation.electrical.electrical\"}],\"Top\":[]}"
      mask Type: simple Variable RL (series or parallel)
  Simscape Component6 : SimscapeComponentBlock  SourceFile=variableRL  ComponentPath=variableRL  ComponentVariants="[\"variableRL\"]"  ComponentVariantNames="[\"variableRL\"]"  ClassName=variableRL  SchemaVersion=1  g=1e-9 1/Ohm  typ=1  i_specify=off  i_priority=None  i=0 A  i_nominal_specify=off  i_nominal_value=1  i_nominal_unit=A  v_specify=off  v_priority=None  v=0 V  v_nominal_specify=off  v_nominal_value=1  v_nominal_unit=V  iL_specify=off  iL_priority=High  iL=0 A  iL_nominal_specify=off  iL_nominal_value=1  iL_nominal_unit=A
      settings: CopyFcn=simscape.engine.sli.internal.componentblockcallback(gcbh,'COPY')  PreCopyFcn=simscape.engine.sli.internal.componentblockcallback(gcbh,'PRECOPY')  PreDeleteFcn=simscape.engine.sli.internal.componentblockcallback(gcbh,'PREDELETE')  InternalSimscapePortConfiguration="{\"Bottom\":[],\"Left\":[{\"id\":\"p\",\"label\":\"+\",\"type\":\"foundation.electrical.electrical\"},{\"id\":\"L\",\"label\":\"L\",\"type\":\"input\"},{\"id\":\"R\",\"label\":\"R\",\"type\":\"input\"}],\"Right\":[{\"id\":\"n\",\"label\":\"-\",\"type\":\"foundation.electrical.electrical\"}],\"Top\":[]}"
      mask Type: simple Variable RL (series or parallel)
  Simulink-PS Converter{,1..14} (15 alike) : nesl_utility/Simulink-PS Converter  PhysicalDomain=network_engine_domain  SubClassName=ps_input  LeftPortType=input  RightPortType=output  PseudoPeriodic=off  Frequencies=[]  NoiseDistribution=none  NoiseParameters=[]  Unit=1  AffineConversion=off  FilteringAndDerivatives=provide  SimscapeFilterOrder=1  InputFilterTimeConstant=0.001  UdotUserProvided=0
  Variable Capacitor : ee_lib/Passive/Variable Capacitor  prm=2  Cmin=1e-9 F  r=1e-6 Ohm  v0=0 V  q0=0 C
      settings: InternalSimscapePortConfiguration="{\"Bottom\":[],\"Left\":[{\"id\":\"C\",\"label\":\"C\",\"type\":\"input\"},{\"id\":\"p\",\"label\":\"+\",\"type\":\"foundation.electrical.electrical\"}],\"Right\":[{\"id\":\"n\",\"label\":\"-\",\"type\":\"foundation.electrical.electrical\"}],\"Top\":[]}"
  Variable Capacitor1 : ee_lib/Passive/Variable Capacitor  prm=2  Cmin=1e-9 F  r=1e-6 Ohm  v0=0 V  q0=0 C
      settings: InternalSimscapePortConfiguration="{\"Bottom\":[],\"Left\":[{\"id\":\"C\",\"label\":\"C\",\"type\":\"input\"},{\"id\":\"p\",\"label\":\"+\",\"type\":\"foundation.electrical.electrical\"}],\"Right\":[{\"id\":\"n\",\"label\":\"-\",\"type\":\"foundation.electrical.electrical\"}],\"Top\":[]}"
  Variable Capacitor2 : ee_lib/Passive/Variable Capacitor  prm=2  Cmin=1e-9 F  r=1e-6 Ohm  v0=0 V  q0=0 C
      settings: InternalSimscapePortConfiguration="{\"Bottom\":[],\"Left\":[{\"id\":\"C\",\"label\":\"C\",\"type\":\"input\"},{\"id\":\"p\",\"label\":\"+\",\"type\":\"foundation.electrical.electrical\"}],\"Right\":[{\"id\":\"n\",\"label\":\"-\",\"type\":\"foundation.electrical.electrical\"}],\"Top\":[]}"
  ABC : PMIOPort  Side=Right
  abc : PMIOPort  Port=2  Side=Left
  wires:
  [Rx] -> Simulink-PS Converter11/1
  [Ls] -> Simulink-PS Converter13/1
  [Cx] -> Simulink-PS Converter12/1
  [Lx] -> Simulink-PS Converter10/1
  [Rs] -> Simulink-PS Converter14/1
  [Rs] -> Simulink-PS Converter9/1
  [Lx] -> Simulink-PS Converter5/1
  [Cx] -> Simulink-PS Converter7/1
  [Ls] -> Simulink-PS Converter8/1
  [Rx] -> Simulink-PS Converter6/1
  Rs/1 -> [Rs]
  Lx/1 -> [Lx]
  Rx/1 -> [Rx]
  Cx/1 -> [Cx]
  [Rx] -> Simulink-PS Converter1/1
  [Ls] -> Simulink-PS Converter3/1
  [Cx] -> Simulink-PS Converter2/1
  [Lx] -> Simulink-PS Converter/1
  Ls/1 -> [Ls]
  [Rs] -> Simulink-PS Converter4/1
  connections:
  Variable Capacitor1/LConn2 -- Phase Splitter/RConn2 -- Simscape Component3/LConn1
  Simulink-PS Converter12/RConn1 -- Variable Capacitor2/LConn1
  Simulink-PS Converter11/RConn1 -- Simscape Component5/LConn3
  Simulink-PS Converter13/RConn1 -- Simscape Component6/LConn2
  Simulink-PS Converter14/RConn1 -- Simscape Component6/LConn3
  Simulink-PS Converter10/RConn1 -- Simscape Component5/LConn2
  Simscape Component6/LConn1 -- Variable Capacitor2/RConn1 -- Simscape Component5/RConn1
  Phase Splitter/RConn3 -- Variable Capacitor2/LConn2 -- Simscape Component5/LConn1
  Simulink-PS Converter7/RConn1 -- Variable Capacitor1/LConn1
  Simulink-PS Converter5/RConn1 -- Simscape Component3/LConn2
  Simulink-PS Converter6/RConn1 -- Simscape Component3/LConn3
  Simulink-PS Converter9/RConn1 -- Simscape Component4/LConn3
  Simulink-PS Converter8/RConn1 -- Simscape Component4/LConn2
  Variable Capacitor1/RConn1 -- Simscape Component4/LConn1 -- Simscape Component3/RConn1
  Simulink-PS Converter3/RConn1 -- Simscape Component2/LConn2
  Simulink-PS Converter4/RConn1 -- Simscape Component2/LConn3
  Simscape Component2/LConn1 -- Variable Capacitor/RConn1 -- Simscape Component1/RConn1
  Simulink-PS Converter1/RConn1 -- Simscape Component1/LConn3
  Simulink-PS Converter/RConn1 -- Simscape Component1/LConn2
  Simscape Component6/RConn1 -- Phase Splitter1/RConn3
  Simscape Component4/RConn1 -- Phase Splitter1/RConn2
  Simscape Component2/RConn1 -- Phase Splitter1/RConn1
  ABC/RConn1 -- Phase Splitter1/LConn1
  abc/RConn1 -- Phase Splitter/LConn1
  Simulink-PS Converter2/RConn1 -- Variable Capacitor/LConn1
  Simscape Component1/LConn1 -- Phase Splitter/RConn1 -- Variable Capacitor/LConn2

== system station2a/Subsystem ==
  In1 : Inport
  Discrete Monostable1 : powerlib_extras/Discrete  Control Blocks/Discrete Monostable  EdgeDetect=Falling  t_mono=0.1  ic=0  Ts=Ts
  Logical Operator1 : Logic  Operator=NOT  AllPortsSameDT=off  OutDataTypeStr=boolean
  commfault : Subsystem
  Out1 : Outport
  wires:
  In1/1 -> commfault/1(In1)
  Logical Operator1/1 -> Out1/1
  commfault/1(Out1) -> Discrete Monostable1/1
  Discrete Monostable1/1 -> Logical Operator1/1

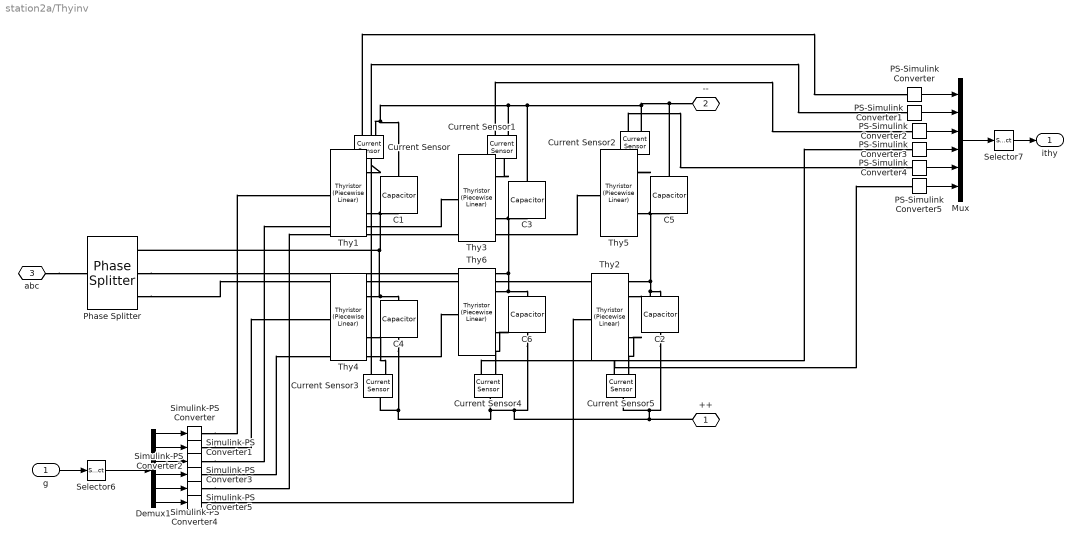
== system station2a/Thyinv ==
  g : Inport
  C{1..6} (6 alike) : ee_lib/Passive/Capacitor  cap_option=ee.enum.passive.capacitor.capOption.const  c=Csnu F  Cvec=[1e-05, 1e-06] F  Vvec=[0, 10] V  CV_table_symmetry=ee.enum.passive.capacitor.tableSymmetry.yes  f_vec=[1, 10] kHz  DFext_vec=[.8, 1.2]  enable_C_tol=ee.enum.toleranceApplication.none  averaging_period=0 s  C_tol=5  tol_distribution=ee.enum.toleranceDistribution.uniform  nSigma=4  r=Rsnu Ohm  g=0 1/Ohm  enable_operating_limits=ee.enum.enable.no  operating_limit_action=ee.enum.passive.reportOpLim.warn  max_working_voltage_range=[-25, 25] V  power_rating=1 W  maxTemperature=85 degC  thermalEnable=false  thermalMass=1 J/K  fault_action=simscape.enum.assert.action.none  t_fault=1 s  i_specify=off  i_priority=None  i=0 A  i_nominal_specify=off  i_nominal_value=1  i_nominal_unit=A  v_specify=off  v_priority=None  v=0 V  v_nominal_specify=off  v_nominal_value=1  v_nominal_unit=V  vc_specify=off  vc_priority=High  vc=0 V  vc_nominal_specify=off  vc_nominal_value=1  vc_nominal_unit=V  T_specify=off  T_priority=None  T=298.15 K  T_nominal_specify=off  T_nominal_value=1  T_nominal_unit=K
  Current Sensor{,1..5} (6 alike) : fl_lib/Electrical/Electrical Sensors/Current Sensor
  Demux1 : Demux  Outputs=6
  Mux : Mux  Inputs=6
  PS-Simulink Converter{,1..5} (6 alike) : nesl_utility/PS-Simulink Converter  PhysicalDomain=network_engine_domain  SubClassName=ps_output  LeftPortType=input  RightPortType=output  PseudoPeriodic=off  Frequencies=[]  VectorFormat=inherit  Unit=inherit  AffineConversion=off
  Phase Splitter : ee_lib/Connectors & References/Phase Splitter
  Selector6 : Selector  InputPortWidth=6  IndexOptions=Index vector (dialog)  Indices=[1 4 3 6 5 2]  OutputSizes=1
  Selector7 : Selector  InputPortWidth=6  IndexOptions=Index vector (dialog)  Indices=[1 6 3 2 5 4]  OutputSizes=1
  Simulink-PS Converter{,1..5} (6 alike) : nesl_utility/Simulink-PS Converter  PhysicalDomain=network_engine_domain  SubClassName=ps_input  LeftPortType=input  RightPortType=output  PseudoPeriodic=off  Frequencies=[]  NoiseDistribution=none  NoiseParameters=[]  Unit=1  AffineConversion=off  FilteringAndDerivatives=provide  SimscapeFilterOrder=1  InputFilterTimeConstant=0.001  UdotUserProvided=0
  Thy{1..6} (6 alike) : ee_lib/Semiconductors & Converters/Thyristor (Piecewise Linear)  port_option=ee.enum.controlport.ps  Vf=0.8 V  Ron=0.001 Ohm  Goff=1e-5 1/Ohm  Vgt=0.5 V  Ih=1 A  diode_param=ee.enum.semiconductors.protectionDiode.external  diode_Vf=0.8 V  diode_Ron=0.001 Ohm  diode_Goff=1e-5 1/Ohm  diode_C=50e-9 F  diode_iRM=-235 A  diode_iF=300 A  diode_idot=-50 A/us  diode_trr_param=ee.enum.converters.diodetrr.trr_factor  diode_trr_factor=3  diode_trr=15 us  diode_Qrr=1500 s*uA  iak_specify=off  iak_priority=None  iak=0 A  iak_nominal_specify=off  iak_nominal_value=1  iak_nominal_unit=A  vak_specify=off  vak_priority=None  vak=0 V  vak_nominal_specify=off  vak_nominal_value=1  vak_nominal_unit=V  vgk_specify=off  vgk_priority=None  vgk=0 V  vgk_nominal_specify=off  vgk_nominal_value=1  vgk_nominal_unit=V  thermal_loss_option=ee.enum.converters.thermalLossOption.constantvalues  Von_data=[0, .1, .6, .8, 1, 1.3, 1.6, 2, 2.4; 0, .1, .7, 1, 1.2, 1.5, 1.9, 2.4, 2.8] V  Tj=[298.15, 398.15] K  Iout_data=[0, .1, 1, 5, 10, 20, 40, 70, 100] A  Eon_data=[0, .0024, .024, .12, .2, .48, 1.04, 2.16, 3.24; 0, .003, .03, .15, .25, .6, 1.3, 2.7, 4.05] * 1e-3 J  Tj_loss=[298.15, 398.15] K  Iout_data_loss=[0, .1, 1, 5, 10, 20, 40, 70, 100] A  Eon_scalar=22.86e-3 J  Eoff_natural_commutation=10e-3 J  Voff=300 V  Iout_scalar=600 A  onCurrentMeasDelay=1e-4 s  diodeModelType=ee.enum.converters.diodeModelType.pwl  diodeTableType=ee.enum.diode.tableType.IfMat  diode_IfMat=[.07, .12, .19, 1.75, 4.24, 7.32, 11.2; .16, .3, .72, 2.14, 4.02, 6.35, 9.12] A  diode_VfMat=[.9, 1.15, 1.25, 1.5, 1.75, 2.17, 2.6, 2.85; .58, .68, .75, 1.1, 1.38, 1.77, 2.27, 2.7] V  diode_TjVec=[25, 125] degC  diode_VfVec=[.5, .7, .9, 1.3, 1.7, 2.1, 2.5] V  diode_IfVec=[.1, .2, .5, 1, 2, 4, 7, 10] A  diode_rec_loss_model=ee.enum.diode.reverseRecoveryModel.fixed  diode_ErecVal=0 J  diode_scaleWithIandV=true  diode_ErecMat=zeros(2, 3) J  diode_TjrecVec=[298.15, 398.15] K  diode_IfrecVec=[.1, 1, 10] A  diode_IrecVal=10 A  diode_VrecVal=10 V  diode_tFilter=1 / 1000 / 100 s  thermal_network_parameterization=ee.enum.thermalNetworkTopology.external  Rth=[.08, .5] K/W  Rth_Cauer=[.08, .1, .5] K/W  Rth_Foster=[.08, .14, .22, .16] K/W  thermal_mass_parameterization=ee.enum.thermalNetwork.timeconstant  thermal_mass=[.01, .5] J/K  thermal_mass_Cauer=[.01, .1, .5] J/K  thermal_mass_Foster=[.001, .005, .05, .5] J/K  thermal_time_constant=[.001, .2] s  thermal_time_constant_Cauer=[.001, .1, .2] s  thermal_time_constant_Foster=[7e-05, .0007, .01, .08] s  thermal_mass_initial_temperatures=[25, 25] degC  thermal_mass_initial_temperatures_Cauer=[25, 25, 25] degC  junction_thermal_mass=0.01 J/K  Tvec_initial_Foster=[25, 25, 25, 25] degC  junction_temperature_specify=off  junction_temperature_priority=None  junction_temperature=25 degC  junction_temperature_nominal_specify=off  junction_temperature_nominal_value=1  junction_temperature_nominal_unit=degC  Qj_specify=off  Qj_priority=None  Qj=0 W  Qj_nominal_specify=off  Qj_nominal_value=1  Qj_nominal_unit=W  accumulatedSwitchingLosses_specify=off  accumulatedSwitchingLosses_priority=None  accumulatedSwitchingLosses=0 J
      settings: InternalSimscapePortConfiguration="{\"Bottom\":[],\"Left\":[{\"id\":\"G\",\"label\":\"\",\"type\":\"input\"}],\"Right\":[{\"id\":\"A\",\"label\":\"\",\"type\":\"foundation.electrical.electrical\"},{\"id\":\"K\",\"label\":\"\",\"type\":\"foundation.electrical.electrical\"}],\"Top\":[]}"
  ++ : PMIOPort  Side=Right
  -- : PMIOPort  Port=2  Side=Right
  abc : PMIOPort  Port=3  Side=Left
  ithy : Outport
  wires:
  PS-Simulink Converter5/1 -> Mux/6
  PS-Simulink Converter4/1 -> Mux/5
  PS-Simulink Converter3/1 -> Mux/4
  PS-Simulink Converter2/1 -> Mux/3
  PS-Simulink Converter1/1 -> Mux/2
  PS-Simulink Converter/1 -> Mux/1
  Mux/1 -> Selector7/1
  Selector7/1 -> ithy/1
  Demux1/5 -> Simulink-PS Converter4/1
  Demux1/4 -> Simulink-PS Converter3/1
  Demux1/1 -> Simulink-PS Converter/1
  Demux1/3 -> Simulink-PS Converter2/1
  Demux1/6 -> Simulink-PS Converter5/1
  Demux1/2 -> Simulink-PS Converter1/1
  Selector6/1 -> Demux1/1
  g/1 -> Selector6/1
  connections:
  Current Sensor5/RConn1 -- PS-Simulink Converter5/LConn1
  Current Sensor2/RConn1 -- PS-Simulink Converter4/LConn1
  Current Sensor4/RConn1 -- PS-Simulink Converter3/LConn1
  Current Sensor1/RConn1 -- PS-Simulink Converter2/LConn1
  Current Sensor3/RConn1 -- PS-Simulink Converter1/LConn1
  Current Sensor/RConn1 -- PS-Simulink Converter/LConn1
  Thy2/RConn1 -- Current Sensor5/RConn2
  Thy6/RConn1 -- Current Sensor4/RConn2
  C6/RConn1 -- C2/RConn1 -- Current Sensor5/LConn1 -- ++/RConn1 -- Current Sensor4/LConn1 -- C4/RConn1 -- Current Sensor3/LConn1
  Thy4/RConn1 -- Current Sensor3/RConn2
  Thy5/RConn2 -- Current Sensor2/LConn1
  Thy3/RConn2 -- Current Sensor1/LConn1
  Thy1/RConn2 -- Current Sensor/LConn1
  abc/RConn1 -- Phase Splitter/LConn1
  Simulink-PS Converter5/RConn1 -- Thy2/LConn1
  Simulink-PS Converter4/RConn1 -- Thy5/LConn1
  Simulink-PS Converter3/RConn1 -- Thy6/LConn1
  Simulink-PS Converter2/RConn1 -- Thy3/LConn1
  Simulink-PS Converter1/RConn1 -- Thy4/LConn1
  Simulink-PS Converter/RConn1 -- Thy1/LConn1
  Phase Splitter/RConn2 -- Thy3/RConn1 -- C3/RConn1 -- Thy6/RConn2 -- C6/LConn1
  C3/LConn1 -- Current Sensor2/RConn2 -- --/RConn1 -- C5/LConn1 -- C1/LConn1 -- Current Sensor/RConn2 -- Current Sensor1/RConn2
  Phase Splitter/RConn3 -- Thy5/RConn1 -- C5/RConn1 -- C2/LConn1 -- Thy2/RConn2
  Phase Splitter/RConn1 -- Thy1/RConn1 -- C1/RConn1 -- Thy4/RConn2 -- C4/LConn1
